simulink model "pll_2"  (R2016a)
settings: Solver=VariableStepAuto  StartTime=0.0  StopTime=2500  RelTol=1e-3
undefined symbols (not defined in the file or in its folder): jsin
libraries: dspsrcs4 x1
settings Model: Creator=coltmt  LastModifiedBy=coltmt
settings DataIOCC: LimitDataPoints=on
settings DebuggingCC: AllowSymbolicDim=off
settings ModelReferenceCC: PropagateSignalLabelsOutOfModel=off
settings GRTTargetCC: GeneratePreprocessorConditionals=Use local settings

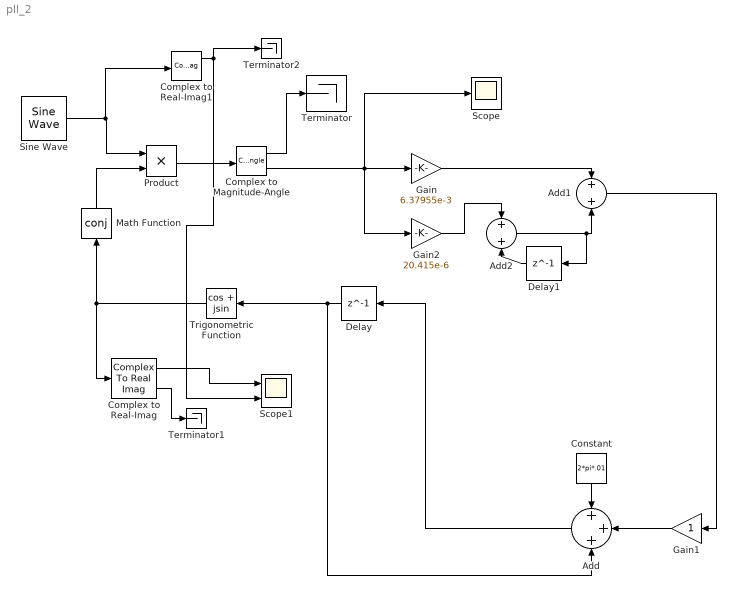
== system pll_2 ==
  Add : Sum  Inputs=+++
  Add1 : Sum
  Add2 : Sum
  Complex to Magnitude-Angle : ComplexToMagnitudeAngle
  Complex to Real-Imag : ComplexToRealImag
  Complex to Real-Imag1 : ComplexToRealImag
  Constant : Constant  Value=2*pi*.01
  Delay : Delay  DelayLength=1
  Delay1 : Delay  DelayLength=1
  Gain : Gain  Gain=6.37955e-3
  Gain1 : Gain
  Gain2 : Gain  Gain=20.415e-6
  Math Function : Math  Operator=conj  SaturateOnIntegerOverflow=on
  Product : Product
  Scope : Scope
  Scope1 : Scope  NumInputPorts=2
  Sine Wave : dspsrcs4/Sine Wave  Amplitude=1  Frequency=.0105  Phase=pi  SampleMode=Discrete  OutComplex=Complex  CompMethod=Trigonometric fcn  TableSize=Speed  SampleTime=1  SamplesPerFrame=1  ResetState=Restart at time zero  OutputFrames=on  dataType=double  wordLen=16  udDataType=sfix(16)  fracBitsMode=Best precision  numFracBits=15  OutDataTypeStr=double  LastOutDataTypeStr=double
  Terminator : Terminator
  Terminator1 : Terminator
  Terminator2 : Terminator
  Trigonometric Function : Trigonometry  Operator=cos + jsin
  wires:
  Constant/1 -> Add/1
  Add/1 -> Delay/1
  Delay/1 -> Trigonometric Function/1, Add/3
  Product/1 -> Complex to Magnitude-Angle/1
  Complex to Magnitude-Angle/1 -> Terminator/1
  Complex to Magnitude-Angle/2 -> Gain2/1, Gain/1, Scope/1
  Math Function/1 -> Product/2
  Sine Wave/1 -> Complex to Real-Imag1/1, Product/1
  Gain1/1 -> Add/2
  Trigonometric Function/1 -> Math Function/1, Complex to Real-Imag/1
  Complex to Real-Imag/1 -> Scope1/1
  Complex to Real-Imag/2 -> Terminator1/1
  Complex to Real-Imag1/1 -> Scope1/2, Terminator2/1
  Gain/1 -> Add1/1
  Delay1/1 -> Add2/2
  Add2/1 -> Delay1/1, Add1/2
  Gain2/1 -> Add2/1
  Add1/1 -> Gain1/1
